simulink model "sm_boom_lift_crawler_test_extend_hydr"  (R2026a)
settings: Solver=ode23t  StopTime=tVec.StopTime  AbsTol=1e-3
PostLoadFcn:
  | sm_boom_lift_crawler_settest('extend only test')
StartFcn:
  | tic;
StopFcn:
  | Elapsed_Sim_Time = toc;
  | %disp(['Elapsed Sim Time = ' num2str(Elapsed_Sim_Time)]);
undefined symbols (not defined in the file): motion, oVec, tVec, X, Y, Z
libraries: nesl_utility x6, sm_boom_lift_crawler_lib x5, sm_lib x5, sm_boom_lift_crawler_lib_boom x2, simulink_extras x2, sm_boom_lift_crawler_lib_actuators x1, sm_boom_lift_crawler_lib_inputs x1, fl_lib x1
Description:
  | Copyright 2025-2026 The MathWorks, Inc.
settings Model: Creator=smiller  LastModifiedBy=smiller
settings DataIOCC: SignalLoggingName=logsout_sm_boom_lift_crawler
settings SimscapeCC: SimscapeNominalValues="[{\"value\":\"1\",\"unit\":\"A\"},{\"value\":\"nomval_psi\",\"unit\":\"psi\"},{\"value\":\"1\",\"unit\":\"cm^2\"},{\"value\":\"nomval_cmv3_s\",\"unit\":\"cm^3/s\"},{\"value\":\"1\",\"unit\":\"kJ/kg\"},{\"value\":\"1\",\"unit\":\"kW\"},{\"value\":\"1\",\"unit\":\"l\"},{\"value\":\"nomval_N\",\"unit\":\"N\"},{\"value\":\"nomval_Nm\",\"unit\":\"N*m\"},{\"value\":\"1\",\"unit\":\"V\"}]"  SimscapeLogName=simlog_sm_boom_lift_crawler  SimscapeLogLimitData=off  SimscapeLogDataHistory=5000.0
settings DiagnosticsConfigSet: SimMechanicsConflictingReferenceFrames=none  SimMechanicsRigidlyBoundBlock=none
settings ExplorerConfigSet: InternalSimMechanicsExplorerSettings="<ExplorerConfiguration><canonicalview>default</canonicalview><AnimationSetting><BasePlaybackSpeed>1.0</BasePlaybackSpeed><PlaybackSpeedFactor>8.0</PlaybackSpeedFactor></AnimationSetting><TilePanel><TileInfo><Tiles Columns=\"1\" Count=\"1\" Rows=\"1\"><Column Weight=\"1\"/><Row Weight=\"1\"/><Tile Height=\"1\" Width=\"1\" X=\"0\" Y=\"0\"/></Tiles></TileInfo><SceneInfo><SceneViewer><BGColor><R>1</R><G>1</G><B>1</B></BGColor><Camera><DoPerspective>on</DoPerspective><Position><X>-0.461900000000000865</X><Y>-2.50030948877568626</Y><Z>1.72278294247342978</Z></Position><Center><X>0.0380999999999989125</X><Y>-1.63477987402602798</Y><Z>1.75208287406564334</Z></Center><Up><X>-5.6968318951078345e-15</X><Y>-0.0338326467840008999</Y><Z>0.999427512134616558</Z></Up><ViewLimDist>1</ViewLimDist><YLim>0.466307658154998583</YLim><XLim>0.590197515672193807</XLim></Camera></SceneViewer></SceneInfo></TilePanel><MechEditorPanel><Cameras><Camera><Id>Camera8</Id><Value><Name>Extend_Knuckle</Name><NativeCamera><PositionTrackingFeature>Boom.Telescope.Extend_Cylinder.Transform_Camera_Extend_Knuckle.F</PositionTrackingFeature><CenterTrackingFeature>Boom.Telescope.Extend_Cylinder.Transform_Camera_Extend_Knuckle.F</CenterTrackingFeature><UpVectorTrackingFeature>Boom.Telescope.Extend_Cylinder.Transform_Camera_Extend_Knuckle.F</UpVectorTrackingFeature><CenterTrackingOrigin>off</CenterTrackingOrigin><CenterTrackingDirection>-X</CenterTrackingDirection><UpVectorTrackingDirection>-Y</UpVectorTrackingDirection></NativeCamera></Value></Camera><Camera><Id>Camera9</Id><Value><Name>Extend_Basket</Name><NativeCamera><PositionTrackingFeature>Boom.Telescope.Extend_Cylinder.Transform_Camera_Extend_Basket.F</PositionTrackingFeature><CenterTrackingFeature>Boom.Telescope.Extend_Cylinder.Transform_Camera_Extend_Basket.F</CenterTrackingFeature><UpVectorTrackingFeature>Boom.Telescope.Extend_Cylinder.Transform_Camera_Extend_Basket.F</UpVectorTrackingFeature><CenterTrackingOrigin>off</CenterTrackingOrigin><CenterTrackingDirection>+X</CenterTrackingDirection><UpVectorTrackingDirection>+Y</UpVectorTrackingDirection></NativeCamera></Value></Camera><Camera><Id>Camera10</Id><Value><Name>Basket_Rotate</Name><NativeCamera><PositionTrackingFeature>Boom.Basket.Basket_Rotate.Bracket.Reference_Camera_Basket_Rotate_L.R</PositionTrackingFeature><CenterTrackingFeature>Boom.Basket.Basket_Rotate.Bracket.Reference_Camera_Basket_Rotate_L.R</CenterTrackingFeature><UpVectorTrackingFeature>Boom.Basket.Basket_Rotate.Bracket.Reference_Camera_Basket_Rotate_L.R</UpVectorTrackingFeature><CenterTrackingOrigin>off</CenterTrackingOrigin><CenterTrackingDirection>-X</CenterTrackingDirection><UpVectorTrackingDirection>+Z</UpVectorTrackingDirection></NativeCamera></Value></Camera><Camera><Id>Camera12</Id><Value><Name>Full Test</Name><NativeCamera><PositionKeyframeSet><Keyframe><Time>0</Time><Value><X>-12.242458171438994</X><Y>-0.1433452642095574</Y><Z>4.1505972342390427</Z></Value></Keyframe><Keyframe><Time>69.026826430124729</Time><Value><X>-14.974593328379619</X><Y>0.0056652615564253064</Y><Z>5.3389029552684786</Z></Value></Keyframe><Keyframe><Time>110.29539843687829</Time><Value><X>-21.00761369699504</X><Y>-0.0057417156870510078</Y><Z>8.0689402037867488</Z></Value></Keyframe><Keyframe><Time>140.70430157635164</Time><Value><X>-31.272784439198116</X><Y>-2.5583130214499052e-10</Y><Z>12.723321478963756</Z></Value></Keyframe><Keyframe><Time>181.77628976806102</Time><Value><X>-31.272784439198116</X><Y>-2.5583130214499052e-10</Y><Z>12.723321478963756</Z></Value></Keyframe><Keyframe><Time>208.0087867386398</Time><Value><X>-23.351505250921551</X><Y>-2.5583182919801497e-10</Y><Z>9.1371534281977738</Z></Value></Keyframe><Keyframe><Time>243.06358572448306</Time><Value><X>-16.577121762622586</X><Y>-2.5583144573665537e-10</Y><Z>6.0702143126734844</Z></Value></Keyframe><Keyframe><Time>273.3415757110605</Time><Value><X>-16.577121762622586</X><Y>-2.5583144573665537e-10</Y><Z>6.0702143126734844</Z></Value></Keyframe><Keyframe><Time>321.2447002217541</Time><Value><X>-13.690590902490033</X><Y>0.01787769923724114</Y><Z>4.7891626503614262</Z></Value></Keyframe><Keyframe><Time>350</Time><Value><X>-13.690590902490033</X><Y>0.01787769923724114</Y><Z>4.7891626503614262</Z></Value></Keyframe></PositionKeyframeSet><CenterKeyframeSet><Keyframe><Time>0</Time><Value><X>-4.621228999686064</X><Y>-0.1433452642095574</Y><Z>4.1505972342390436</Z></Value></Keyframe><Keyframe><Time>69.026826430124729</Time><Value><X>-0.17395018713353672</X><Y>0.0056652615564253064</Y><Z>5.3389029552684786</Z></Value></Keyframe><Keyframe><Time>110.29539843687829</Time><Value><X>-9.0038066291239502</X><Y>-0.0057417156870549491</Y><Z>8.0689402037867524</Z></Value></Keyframe><Keyframe><Time>140.70430157635164</Time><Value><X>-14.136391845814327</X><Y>-2.5583979379462107e-10</Y><Z>12.72332147896376</Z></Value></Keyframe><Keyframe><Time>181.77628976806102</Time><Value><X>-2.3429975002054775</X><Y>-2.5584563781180217e-10</Y><Z>12.723321478963761</Z></Value></Keyframe><Keyframe><Time>208.0087867386398</Time><Value><X>-10.17575261115104</X><Y>-2.5583801743778167e-10</Y><Z>9.1371534281977755</Z></Value></Keyframe><Keyframe><Time>243.06358572448306</Time><Value><X>-0.54476849060194255</X><Y>-2.5583897563257738e-10</Y><Z>6.0702143126734844</Z></Value></Keyframe><Keyframe><Time>273.3415757110605</Time><Value><X>-0.11057247639663359</X><Y>-2.5583917956089291e-10</Y><Z>6.0702143126734844</Z></Value></Keyframe><Keyframe><Time>321.2447002217541</Time><Value><X>-5.3452949964231387</X><Y>0.017877699237237366</Y><Z>4.7891626503614253</Z></Value></Keyframe><Keyframe><Time>350</Time><Value><X>-5.3452949964231387</X><Y>0.017877699237237366</Y><Z>4.7891626503614253</Z></Value></Keyframe></CenterKeyframeSet><UpVectorKeyframeSet><Keyframe><Time>0</Time><Value><X>0</X><Y>0</Y><Z>1</Z></Value></Keyframe><Keyframe><Time>69.026826430124729</Time><Value><X>0</X><Y>0</Y><Z>1</Z></Value></Keyframe><Keyframe><Time>110.29539843687829</Time><Value><X>0</X><Y>0</Y><Z>1</Z></Value></Keyframe><Keyframe><Time>140.70430157635164</Time><Value><X>0</X><Y>0</Y><Z>1</Z></Value></Keyframe><Keyframe><Time>181.77628976806102</Time><Value><X>-2.0731981129868445e-16</X><Y>1.0273382740432149e-31</Y><Z>1</Z></Value></Keyframe><Keyframe><Time>208.0087867386398</Time><Value><X>1.4663775813922931e-57</X><Y>2.9591920320379324e-42</Y><Z>1</Z></Value></Keyframe><Keyframe><Time>243.06358572448306</Time><Value><X>1.3898401336634517e-57</X><Y>2.9591920320379324e-42</Y><Z>1</Z></Value></Keyframe><Keyframe><Time>273.3415757110605</Time><Value><X>1.3898401336605064e-57</X><Y>2.9591920320379324e-42</Y><Z>1</Z></Value></Keyframe><Keyframe><Time>321.2447002217541</Time><Value><X>1.3198478700492623e-57</X><Y>2.9591920320379324e-42</Y><Z>1</Z></Value></Keyframe><Keyframe><Time>350</Time><Value><X>1.0642863113510858e-16</X><Y>-4.813997747953607e-32</Y><Z>1</Z></Value></Keyframe></UpVectorKeyframeSet></NativeCamera></Value></Camera><Camera><Id>Camera13</Id><Value><Name>View_Basket_World</Name><NativeCamera><PositionTrackingFeature>Boom.Basket.Basket.Reference_Basket_Cam.R</PositionTrackingFeature><CenterTrackingFeature>Mech_Config.World.W</CenterTrackingFeature><UpVectorTrackingFeature>Boom.Basket.Basket.Reference_Basket_Cam.R</UpVectorTrackingFeature><CenterTrackingOrigin>on</CenterTrackingOrigin><UpVectorTrackingDirection>+Y</UpVectorTrackingDirection></NativeCamera></Value></Camera><Camera><Id>Camera15</Id><Value><Name>Extend_Retract_Pulley</Name><NativeCamera><PositionTrackingFeature>Boom.Telescope.Extend_Cylinder.Reference_Camera_Retract_Pulley.R</PositionTrackingFeature><CenterTrackingFeature>Boom.Telescope.Extend_Cylinder.Reference_Camera_Retract_Pulley.R</CenterTrackingFeature><UpVectorTrackingFeature>Boom.Telescope.Extend_Cylinder.Reference_Camera_Retract_Pulley.R</UpVectorTrackingFeature><CenterTrackingOrigin>off</CenterTrackingOrigin><CenterTrackingDirection>+Y</CenterTrackingDirection><UpVectorTrackingDirection>+Z</UpVectorTrackingDirection></NativeCamera></Value></Camera><Camera><Id>Camera16</Id><Value><Name>Extend_Extend_Pulley</Name><NativeCamera><PositionTrackingFeature>Boom.Telescope.Extend_Cylinder.Reference_Camera_Extend_Pulley.R</PositionTrackingFeature><CenterTrackingFeature>Boom.Telescope.Extend_Cylinder.Reference_Camera_Extend_Pulley.R</CenterTrackingFeature><UpVectorTrackingFeature>Boom.Telescope.Extend_Cylinder.Reference_Camera_Extend_Pulley.R</UpVectorTrackingFeature><CenterTrackingOrigin>off</CenterTrackingOrigin><CenterTrackingDirection>+Z</CenterTrackingDirection><UpVectorTrackingDirection>-Y</UpVectorTrackingDirection></NativeCamera></Value></Camera><Camera><Id>Camera17</Id><Value><Name>Jib</Name><NativeCamera><PositionTrackingFeature>Boom.Basket.Jib.Jib_Mount.Reference_Camera_Basket_Jib.R</PositionTrackingFeature><CenterTrackingFeature>Boom.Basket.Jib.Jib_Mount.Reference_Camera_Basket_Jib.R</CenterTrackingFeature><UpVectorTrackingFeature>Mech_Config.World.W</UpVectorTrackingFeature><CenterTrackingOrigin>off</CenterTrackingOrigin><CenterTrackingDirection>-X</CenterTrackingDirection><UpVectorTrackingDirection>+Z</UpVectorTrackingDirection></NativeCamera></Value></Camera></Cameras><GfxPanelCameraMap><MapElement CameraMLId=\"Camera15\" GfxPanelIndex=\"0\"/></GfxPanelCameraMap><VideoCreator><PlaybackSpeedRatio>8</PlaybackSpeedRatio><FrameRate>30</FrameRate><VideoFormat>MPEG-4</VideoFormat><FrameSize>auto</FrameSize></VideoCreator></MechEditorPanel></ExplorerConfiguration>"

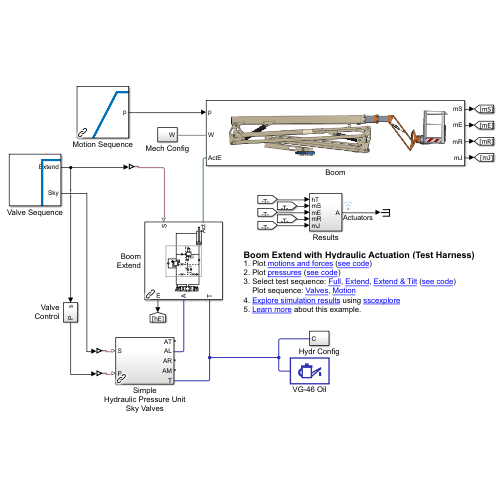
[thumbnail: Simulink's stored preview of the top-level diagram]
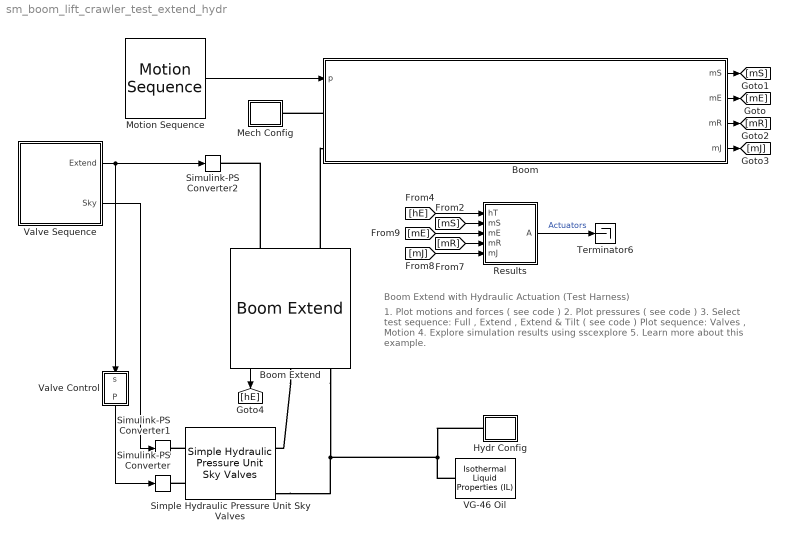
== system sm_boom_lift_crawler_test_extend_hydr ==
  note: 1. Plot motions and forces ( see code )
      | 2. Plot pressures ( see code )
      | 3. Select test sequence: Full , Extend , Extend & Tilt ( see code )
      | Plot sequence: Valves , Motion
      | 4. Explore simulation results using sscexplore
      | 5. Learn more about this example.
  note: Boom Extend with Hydraulic Actuation (Test Harness)
  Boom : Subsystem
      mask Display: image('sm002.svg');
  Boom Extend : sm_boom_lift_crawler_lib_actuators/Actuators/Sky Manifold/Sky Valves II/Boom Extend  SystemSampleTime=-1  VariantActivationTime=update diagram  EmptyChoice=off  PassThrough=off  PassThroughVariantControl=(default)  EmptyChoiceVariantControl=(default)  AllowFlexibleInterface=on  Latency=0  AutoFrameSizeCalculation=off
  Hydr Config : Subsystem
  Mech Config : Subsystem
  Motion Sequence : sm_boom_lift_crawler_lib_inputs/Motion Sequence  SystemSampleTime=-1  VariantActivationTime=update diagram  EmptyChoice=off  PassThrough=off  PassThroughVariantControl=(default)  EmptyChoiceVariantControl=(default)  AllowFlexibleInterface=on  Latency=0  AutoFrameSizeCalculation=off
  Results : Subsystem
  Simple Hydraulic Pressure Unit Sky Valves : sm_boom_lift_crawler_lib/Simple Hydraulic Pressure Unit Sky Valves  SystemSampleTime=-1  VariantActivationTime=update diagram  EmptyChoice=off  PassThrough=off  PassThroughVariantControl=(default)  EmptyChoiceVariantControl=(default)  AllowFlexibleInterface=on  Latency=0  AutoFrameSizeCalculation=off
  Simulink-PS Converter : nesl_utility/Simulink-PS Converter  PhysicalDomain=network_engine_domain  SubClassName=ps_input  LeftPortType=input  RightPortType=output  PseudoPeriodic=off  Frequencies=[]  NoiseDistribution=none  NoiseParameters=[]  Unit=Pa  AffineConversion=off  FilteringAndDerivatives=provide  SimscapeFilterOrder=1  InputFilterTimeConstant=0.001  UdotUserProvided=0
  Simulink-PS Converter1 : nesl_utility/Simulink-PS Converter  PhysicalDomain=network_engine_domain  SubClassName=ps_input  LeftPortType=input  RightPortType=output  PseudoPeriodic=off  Frequencies=[]  NoiseDistribution=none  NoiseParameters=[]  Unit=1  AffineConversion=off  FilteringAndDerivatives=provide  SimscapeFilterOrder=1  InputFilterTimeConstant=0.001  UdotUserProvided=0
  Simulink-PS Converter2 : nesl_utility/Simulink-PS Converter  PhysicalDomain=network_engine_domain  SubClassName=ps_input  LeftPortType=input  RightPortType=output  PseudoPeriodic=off  Frequencies=[]  NoiseDistribution=none  NoiseParameters=[]  Unit=1  AffineConversion=off  FilteringAndDerivatives=provide  SimscapeFilterOrder=1  InputFilterTimeConstant=0.001  UdotUserProvided=0
  Terminator6 : Terminator
  VG-46 Oil : fl_lib/Isothermal Liquid/Utilities/Isothermal Liquid Properties (IL)  rho_L_atm=867.346 kg/m^3  bulk_modulus_model=foundation.enum.bulk_modulus_model.const  beta_gain=6  beta_L_atm=1.48150e+09 Pa  nu_atm=(45.7333)*(1) cSt  p_atm=0.101325 MPa  p_min=1 Pa  properties_range_check=simscape.enum.assert.action.error  air_fraction=ratio_dissolved_air  polytropic_index=1.0  rho_g_atm=1.225 kg/m^3  air_dissolution_model=simscape.enum.onoff.off  p_crit=3 MPa
  Valve Control : Subsystem
  Valve Sequence : Subsystem
      mask Display: image('sm_boom_lift_crawler_valve_seq_outputonly.svg');
  wires:
  [mJ] -> Results/5(mJ)
  Boom/2(mE) -> [mE]
  Valve Control/1(P) -> Simulink-PS Converter/1
  [mR] -> Results/4(mR)
  [mE] -> Results/3(mE)
  [hE] -> Results/1(hT)
  Boom/3(mR) -> [mR]
  Results/1(A) -> Terminator6/1  "Actuators"
  Motion Sequence/1 -> Boom/1(p)
  Boom/1(mS) -> [mS]
  Boom Extend/1 -> [hE]
  Boom/4(mJ) -> [mJ]
  Valve Sequence/1(Extend) -> Simulink-PS Converter2/1, Valve Control/1(s)
  Valve Sequence/2(Sky) -> Simulink-PS Converter1/1
  [mS] -> Results/2(mS)
  connections:
  VG-46 Oil/RConn1 -- Hydr Config/RConn1 -- Boom Extend/RConn2 -- Simple Hydraulic Pressure Unit Sky Valves/RConn5
  Simple Hydraulic Pressure Unit Sky Valves/LConn1 -- Simulink-PS Converter1/RConn1
  Boom/LConn1 -- Mech Config/LConn1
  Boom Extend/LConn1 -- Simulink-PS Converter2/RConn1
  Boom Extend/LConn2 -- Boom/LConn2
  Boom Extend/RConn1 -- Simple Hydraulic Pressure Unit Sky Valves/RConn2
  Simple Hydraulic Pressure Unit Sky Valves/LConn2 -- Simulink-PS Converter/RConn1

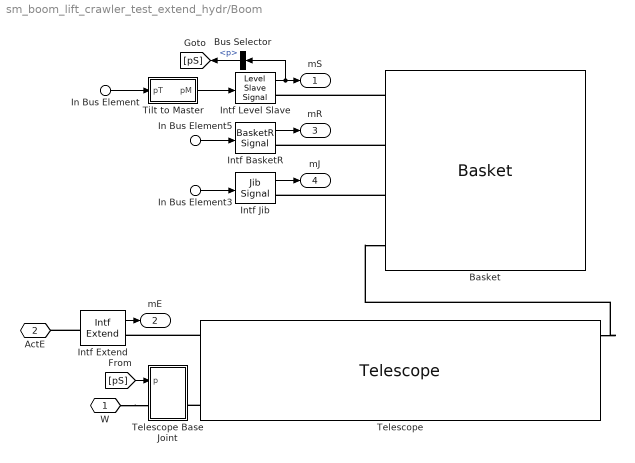
== system sm_boom_lift_crawler_test_extend_hydr/Boom ==
  In Bus Element5 : Inport  PortName=p  Element=BasketR
  In Bus Element3 : Inport  PortName=p  Element=Jib
  In Bus Element : Inport  PortName=p  Element=Tilt
  Basket : sm_boom_lift_crawler_lib_boom/Boom/Basket  SystemSampleTime=-1  VariantActivationTime=update diagram  EmptyChoice=off  PassThrough=off  PassThroughVariantControl=(default)  EmptyChoiceVariantControl=(default)  AllowFlexibleInterface=on  Latency=0  AutoFrameSizeCalculation=off
  Bus Selector : BusSelector  OutputSignals=p
  Intf BasketR : sm_boom_lift_crawler_lib/BasketR Signal  SystemSampleTime=-1  VariantActivationTime=update diagram  EmptyChoice=off  PassThrough=off  PassThroughVariantControl=(default)  EmptyChoiceVariantControl=(default)  AllowFlexibleInterface=on  Latency=0  AutoFrameSizeCalculation=off
  Intf Extend : sm_boom_lift_crawler_lib/Intf Extend  SystemSampleTime=-1  VariantActivationTime=update diagram  EmptyChoice=off  PassThrough=off  PassThroughVariantControl=(default)  EmptyChoiceVariantControl=(default)  AllowFlexibleInterface=on  Latency=0  AutoFrameSizeCalculation=off
  Intf Jib : sm_boom_lift_crawler_lib/Jib Signal  SystemSampleTime=-1  VariantActivationTime=update diagram  EmptyChoice=off  PassThrough=off  PassThroughVariantControl=(default)  EmptyChoiceVariantControl=(default)  AllowFlexibleInterface=on  Latency=0  AutoFrameSizeCalculation=off
  Intf Level Slave : sm_boom_lift_crawler_lib/Level Slave Signal  SystemSampleTime=-1  VariantActivationTime=update diagram  EmptyChoice=off  PassThrough=off  PassThroughVariantControl=(default)  EmptyChoiceVariantControl=(default)  AllowFlexibleInterface=on  Latency=0  AutoFrameSizeCalculation=off
  Telescope : sm_boom_lift_crawler_lib_boom/Boom/Arms/Telescope  SystemSampleTime=-1  VariantActivationTime=update diagram  EmptyChoice=off  PassThrough=off  PassThroughVariantControl=(default)  EmptyChoiceVariantControl=(default)  AllowFlexibleInterface=on  Latency=0  AutoFrameSizeCalculation=off
  Telescope Base Joint : Subsystem
  Tilt to Master : Subsystem
  W : PMIOPort  Side=Left
  ActE : PMIOPort  Port=2  Side=Left
  mS : Outport
  mE : Outport  Port=2
  mR : Outport  Port=3
  mJ : Outport  Port=4
  wires:
  Intf Level Slave/1 -> Bus Selector/1, mS/1
  Intf Extend/1 -> mE/1
  In Bus Element5/1 -> Intf BasketR/1
  In Bus Element3/1 -> Intf Jib/1
  Intf Jib/1 -> mJ/1
  Intf BasketR/1 -> mR/1
  Tilt to Master/1(pM) -> Intf Level Slave/1
  In Bus Element/1 -> Tilt to Master/1(pT)
  Bus Selector/1 -> [pS]  "<p>"
  [pS] -> Telescope Base Joint/1(p)
  connections:
  Basket/RConn2 -- Intf BasketR/RConn1
  Telescope/LConn1 -- Intf Extend/RConn1
  Telescope/LConn3 -- Telescope Base Joint/RConn1
  Telescope/RConn1 -- Basket/RConn4
  Basket/RConn1 -- Intf Level Slave/RConn1
  Basket/RConn3 -- Intf Jib/RConn1
  W/RConn1 -- Telescope Base Joint/LConn1
  Intf Extend/LConn1 -- ActE/RConn1

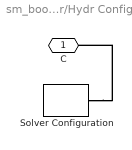
== system sm_boom_lift_crawler_test_extend_hydr/Hydr Config ==
  Solver Configuration : nesl_utility/Solver Configuration  PhysicalDomain=network_engine_domain  SubClassName=solver  LeftPortType=input  RightPortType=generic  Tones=[]  Harmonics=[]  SimulateNoise=off  Profile=off  UseLocalSampling=off  EnableSwitchedLinearOptims=on  FrequencyDomain=off  UseCCode=off  RelTol=0.001  AbsTol=1e-06  MinStep=1e-09  ToWorkspace=off  RevertToSquareIcSolve=off  NumHomotopyIterations=100  PhasorMode=off  PhasorModeNumHarmonics=1  ConsistencySolver=NEWTON_FTOL  CanonicalOrdering=UNORDERED  OptimizeIntermediates=UNOPTIMIZED  IndexReductionMethod=DerivativeReplacement  DoDC=off  ResidualTolerance=1e-9  ConsistencyTolSource=GLOBAL  ConsistencyAbsTol=0.001  ConsistencyRelTol=0.001  ConsistencyTolFactor=0.001  UseLocalSolver=off  LocalSolverChoice=NE_BACKWARD_EULER_ADVANCER  ResolveIndetEquations=on  FunctionEvalNumThread=1  LocalSolverSampleTime=2e-3  DoFixedCost=off  MaxNonlinIter=5  MaxModeIter=2  ComputeImpulses=off  ImpulseIterations=2  LinearAlgebra=Sparse  LinearAlgebraNumThread=0  EquationFormulation=NE_TIME_EF  DelaysMemoryBudget=1024  AutomaticFiltering=on  FilteringTimeConstant=1e-3  PartitionStorageMethod=EXHAUSTIVE  PartitionMemoryBudget=1024  PartitionMethod=FAST  MultibodyUseLocalSolver=off  MultibodyLocalSolverChoice=ODE1  MultibodyLocalSolverSampleTime=0.001
  C : PMIOPort  Side=Right
  connections:
  Solver Configuration/RConn1 -- C/RConn1

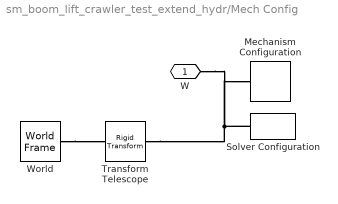
== system sm_boom_lift_crawler_test_extend_hydr/Mech Config ==
  Mechanism Configuration : sm_lib/Utilities/Mechanism Configuration  UniformGravity=Constant  GravityVector=[0 0 -9.80665]  GravityVectorUnits=m/s^2  LinearizationDelta=0.001  JointModeTransitionNonlinearIterations=2
  Solver Configuration : nesl_utility/Solver Configuration  PhysicalDomain=network_engine_domain  SubClassName=solver  LeftPortType=input  RightPortType=generic  Tones=[]  Harmonics=[]  SimulateNoise=off  Profile=off  UseLocalSampling=off  EnableSwitchedLinearOptims=on  FrequencyDomain=off  UseCCode=off  RelTol=0.001  AbsTol=1e-06  MinStep=1e-09  ToWorkspace=off  RevertToSquareIcSolve=off  NumHomotopyIterations=100  PhasorMode=off  PhasorModeNumHarmonics=1  ConsistencySolver=NEWTON_FTOL  CanonicalOrdering=UNORDERED  OptimizeIntermediates=UNOPTIMIZED  IndexReductionMethod=DerivativeReplacement  DoDC=off  ResidualTolerance=1e-9  ConsistencyTolSource=GLOBAL  ConsistencyAbsTol=0.001  ConsistencyRelTol=0.001  ConsistencyTolFactor=0.001  UseLocalSolver=off  LocalSolverChoice=NE_BACKWARD_EULER_ADVANCER  ResolveIndetEquations=on  FunctionEvalNumThread=1  LocalSolverSampleTime=2e-3  DoFixedCost=off  MaxNonlinIter=3  MaxModeIter=2  ComputeImpulses=off  ImpulseIterations=2  LinearAlgebra=auto  LinearAlgebraNumThread=0  EquationFormulation=NE_TIME_EF  DelaysMemoryBudget=1024  AutomaticFiltering=on  FilteringTimeConstant=0.001  PartitionStorageMethod=AS_NEEDED  PartitionMemoryBudget=1024  PartitionMethod=ROBUST  MultibodyUseLocalSolver=off  MultibodyLocalSolverChoice=ODE1  MultibodyLocalSolverSampleTime=0.001
  Transform Telescope : sm_lib/Frames and Transforms/Rigid Transform  RotationMethod=None  FollAlignAxisA=+X  BaseAlignAxisA=+Y  FollAlignAxisB=+Y  BaseAlignAxisB=+Z  RotationStandardAxis=+Z  RotationAngle=0.0  RotationAngleUnits=deg  RotationArbitraryAxis=[0 0 1]  RotationSequenceAxes=FollowerAxes  RotationSequence=XYX  RotationSequenceAngles=[0 0 0]  RotationSequenceAnglesUnits=deg  RotationMatrix=[1 0 0; 0 1 0; 0 0 1]  Quaternion=[1 0 0 0]  TranslationMethod=Cartesian  TranslationCartesianOffset=[-0.1 -3 1.5]  TranslationCartesianOffsetUnits=m  TranslationStandardAxis=+Z  TranslationStandardOffset=0  TranslationStandardOffsetUnits=m  TranslationROffset=0  TranslationROffsetUnits=m  TranslationThetaOffset=0  TranslationThetaOffsetUnits=deg  TranslationZOffset=0  TranslationZOffsetUnits=m
  World : sm_lib/Frames and Transforms/World Frame
  W : PMIOPort  Side=Left
  connections:
  Solver Configuration/RConn1 -- Transform Telescope/RConn1 -- W/RConn1 -- Mechanism Configuration/RConn1
  World/RConn1 -- Transform Telescope/LConn1

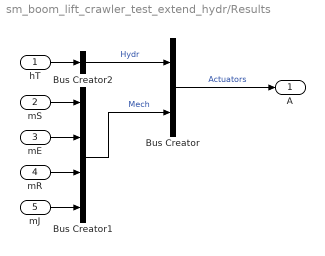
== system sm_boom_lift_crawler_test_extend_hydr/Results ==
  hT : Inport
  mS : Inport  Port=2
  mE : Inport  Port=3
  mR : Inport  Port=4
  mJ : Inport  Port=5
  Bus Creator : BusCreator  Inputs=2
  Bus Creator1 : BusCreator  Inputs=4
  Bus Creator2 : BusCreator  Inputs=1
  A : Outport
  wires:
  hT/1 -> Bus Creator2/1
  Bus Creator/1 -> A/1  "Actuators"
  Bus Creator1/1 -> Bus Creator/2  "Mech"
  Bus Creator2/1 -> Bus Creator/1  "Hydr"
  mS/1 -> Bus Creator1/1
  mE/1 -> Bus Creator1/2
  mR/1 -> Bus Creator1/3
  mJ/1 -> Bus Creator1/4

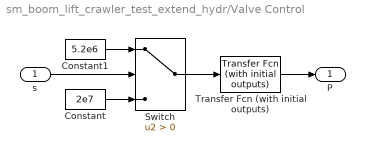
== system sm_boom_lift_crawler_test_extend_hydr/Valve Control ==
  s : Inport
  Constant : Constant  Value=2e7
  Constant1 : Constant  Value=5.2e6
  Switch : Switch  Criteria=u2 > Threshold  SaturateOnIntegerOverflow=off  InputSameDT=off
  Transfer Fcn (with initial outputs) : simulink_extras/Additional Linear/Transfer Fcn (with initial outputs)  N=[1]  D="[0.1  1]"  Y0=2e7  U0=2e7
  P : Outport
  wires:
  Constant/1 -> Switch/3
  Constant1/1 -> Switch/1
  Switch/1 -> Transfer Fcn (with initial outputs)/1
  s/1 -> Switch/2
  Transfer Fcn (with initial outputs)/1 -> P/1

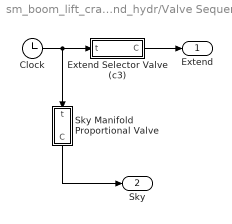
== system sm_boom_lift_crawler_test_extend_hydr/Valve Sequence ==
  Clock : Clock
  Extend Selector Valve (c3) : Subsystem
  Sky Manifold Proportional Valve : Subsystem
  Extend : Outport
  Sky : Outport  Port=2
  wires:
  Clock/1 -> Extend Selector Valve (c3)/1(t), Sky Manifold Proportional Valve/1(t)
  Extend Selector Valve (c3)/1(C) -> Extend/1
  Sky Manifold Proportional Valve/1(C) -> Sky/1

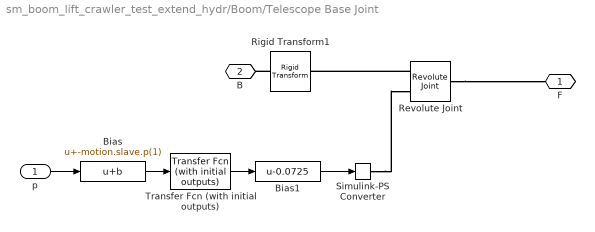
== system sm_boom_lift_crawler_test_extend_hydr/Boom/Telescope Base Joint ==
  p : Inport
  Bias : Bias  Bias=-motion.slave.p(1)  SaturateOnIntegerOverflow=off
  Bias1 : Bias  Bias=-0.0725  SaturateOnIntegerOverflow=off
  Revolute Joint : sm_lib/Joints/Revolute Joint  JointMode=Normal  CompositeWrenchDir=FollowerOnBase  CompositeWrenchFrame=BaseFrame  SenseConstraintForce=off  SenseConstraintTorque=off  SenseTotalForce=off  SenseTotalTorque=off  PositionTargetSpecify=on  PositionTargetPriority=High  PositionTargetValue=-0.0725  PositionTargetValueUnits=deg  VelocityTargetSpecify=off  VelocityTargetPriority=High  VelocityTargetValue=0  VelocityTargetValueUnits=deg/s  EquilibriumPosition=0  EquilibriumPositionUnits=deg  SpringStiffness=0  SpringStiffnessUnits=N*m/deg  DampingCoefficient=0  DampingCoefficientUnits=N*m/(deg/s)  LowerLimitSpecify=off  LowerLimitBound=-90  LowerLimitBoundUnits=deg  LowerLimitStiffness=1e4  LowerLimitStiffnessUnits=N*m/deg  LowerLimitDamping=10  LowerLimitDampingUnits=N*m/(deg/s)  LowerLimitTransitionRegionWidth=0.1  LowerLimitTransitionRegionWidthUnits=deg  UpperLimitSpecify=off  UpperLimitBound=90  UpperLimitBoundUnits=deg  UpperLimitStiffness=1e4  UpperLimitStiffnessUnits=N*m/deg  UpperLimitDamping=10  UpperLimitDampingUnits=N*m/(deg/s)  UpperLimitTransitionRegionWidth=0.1  UpperLimitTransitionRegionWidthUnits=deg  TorqueActuationMode=ComputedTorque  MotionActuationMode=InputMotion  SensePosition=off  SenseVelocity=off  SenseAcceleration=off  SenseTorqueForce=off  SenseLowerLimitTorqueForce=off  SenseUpperLimitTorqueForce=off
  Rigid Transform1 : sm_lib/Frames and Transforms/Rigid Transform  RotationMethod=RotationSequence  FollAlignAxisA=+X  BaseAlignAxisA=+Y  FollAlignAxisB=+Y  BaseAlignAxisB=+Z  RotationStandardAxis=+Y  RotationAngle=-90  RotationAngleUnits=deg  RotationArbitraryAxis=[0 0 1]  RotationSequenceAxes=FollowerAxes  RotationSequence=XYX  RotationSequenceAngles=[-90 90 0]  RotationSequenceAnglesUnits=deg  RotationMatrix=[1 0 0; 0 1 0; 0 0 1]  Quaternion=[1 0 0 0]  TranslationMethod=None  TranslationCartesianOffset=[0 0 0]  TranslationCartesianOffsetUnits=m  TranslationStandardAxis=+Z  TranslationStandardOffset=0  TranslationStandardOffsetUnits=m  TranslationROffset=0  TranslationROffsetUnits=m  TranslationThetaOffset=0  TranslationThetaOffsetUnits=deg  TranslationZOffset=0  TranslationZOffsetUnits=m
  Simulink-PS Converter : nesl_utility/Simulink-PS Converter  PhysicalDomain=network_engine_domain  SubClassName=ps_input  LeftPortType=input  RightPortType=output  PseudoPeriodic=off  Frequencies=[]  NoiseDistribution=none  NoiseParameters=[]  Unit=deg  AffineConversion=off  FilteringAndDerivatives=filter  SimscapeFilterOrder=2  InputFilterTimeConstant=0.1  UdotUserProvided=0
  Transfer Fcn (with initial outputs) : simulink_extras/Additional Linear/Transfer Fcn (with initial outputs)  N=[400]  D="[0.1  1]"  Y0=0  U0=0
  F : PMIOPort  Side=Right
  B : PMIOPort  Port=2  Side=Left
  wires:
  Transfer Fcn (with initial outputs)/1 -> Bias1/1
  p/1 -> Bias/1
  Bias/1 -> Transfer Fcn (with initial outputs)/1
  Bias1/1 -> Simulink-PS Converter/1
  connections:
  Revolute Joint/RConn1 -- F/RConn1
  Rigid Transform1/LConn1 -- B/RConn1
  Simulink-PS Converter/RConn1 -- Revolute Joint/LConn2
  Revolute Joint/LConn1 -- Rigid Transform1/RConn1

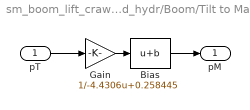
== system sm_boom_lift_crawler_test_extend_hydr/Boom/Tilt to Master ==
  pT : Inport
  Bias : Bias  Bias=0.258445  SaturateOnIntegerOverflow=off
  Gain : Gain  Gain=1/-4.4306
  pM : Outport
  wires:
  Gain/1 -> Bias/1
  pT/1 -> Gain/1
  Bias/1 -> pM/1

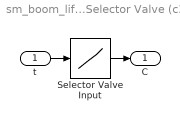
== system sm_boom_lift_crawler_test_extend_hydr/Valve Sequence/Extend Selector Valve (c3) ==
  t : Inport
  Selector Valve Input : Lookup_n-D  NumberOfTableDimensions=1  BreakpointsForDimension1=tVec.sky.c3.all  Table=oVec.sky.c3.all  InterpMethod=Flat  ExtrapMethod=Clip  UseLastTableValue=on  InternalRulePriority=Speed  RndMeth=Simplest
  C : Outport
  wires:
  t/1 -> Selector Valve Input/1
  Selector Valve Input/1 -> C/1

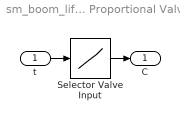
== system sm_boom_lift_crawler_test_extend_hydr/Valve Sequence/Sky Manifold Proportional Valve ==
  t : Inport
  Selector Valve Input : Lookup_n-D  NumberOfTableDimensions=1  BreakpointsForDimension1=tVec.sky.proportional  Table=oVec.sky.proportional  InterpMethod=Flat  ExtrapMethod=Clip  UseLastTableValue=on  InternalRulePriority=Speed  RndMeth=Simplest
  C : Outport
  wires:
  t/1 -> Selector Valve Input/1
  Selector Valve Input/1 -> C/1
